simulink model "Final_Q2_C_end"  (R2019a)
settings: Solver=ode1  StartTime=0.0  StopTime=60  FixedStep=0.01  RelTol=1e-3  EnableMultiTasking=on
settings Model: Creator=enesu  LastModifiedBy=hp
settings SolverCC: AutoInsertRateTranBlk=on

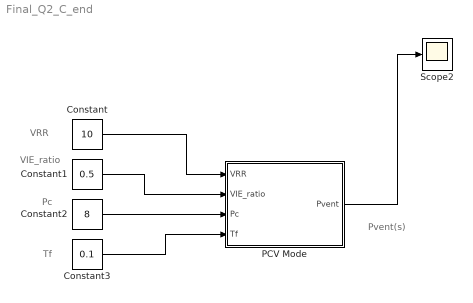
== system Final_Q2_C_end ==
  note: Tf
  note: Pc
  note: VIE_ratio
  note: VRR
  note: Pvent(s)
  Constant : Constant  Value=10  VectorParams1D=off
  Constant1 : Constant  Value=0.5
  Constant2 : Constant  Value=8
  Constant3 : Constant  Value=0.1
  PCV Mode : Subsystem
  Scope2 : Scope
  wires:
  Constant/1 -> PCV Mode/1(VRR)
  Constant1/1 -> PCV Mode/2(VIE_ratio)
  Constant2/1 -> PCV Mode/3(Pc)
  PCV Mode/1(Pvent) -> Scope2/1
  Constant3/1 -> PCV Mode/4(Tf)

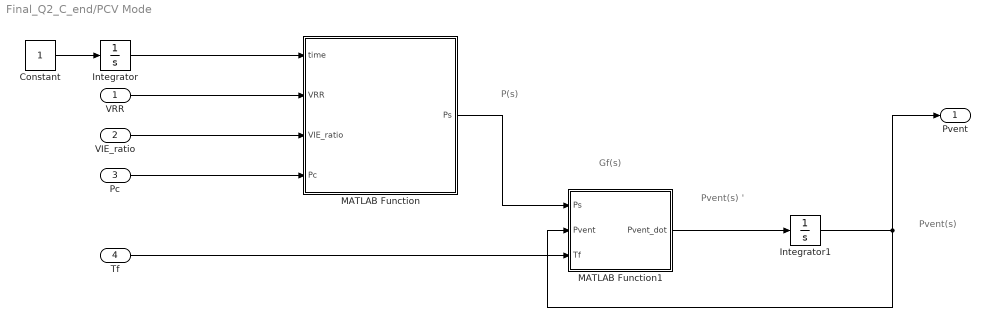
== system Final_Q2_C_end/PCV Mode ==
  note: P(s)
  note: Gf(s)
  note: Pvent(s) '
  note: Pvent(s)
  VRR : Inport
  VIE_ratio : Inport  Port=2
  Pc : Inport  Port=3
  Tf : Inport  Port=4
  Constant : Constant
  Integrator : Integrator
  Integrator1 : Integrator
  MATLAB Function : MATLAB Function  TreatAsAtomicUnit=on
  MATLAB Function1 : MATLAB Function  TreatAsAtomicUnit=on
  Pvent : Outport  VectorParamsAs1DForOutWhenUnconnected=on
  wires:
  Constant/1 -> Integrator/1
  Integrator/1 -> MATLAB Function/1(time)
  VRR/1 -> MATLAB Function/2(VRR)
  VIE_ratio/1 -> MATLAB Function/3(VIE_ratio)
  Pc/1 -> MATLAB Function/4(Pc)
  Tf/1 -> MATLAB Function1/3(Tf)
  MATLAB Function/1(Ps) -> MATLAB Function1/1(Ps)
  MATLAB Function1/1(Pvent_dot) -> Integrator1/1
  Integrator1/1 -> Pvent/1, MATLAB Function1/2(Pvent)

== matlab function Final_Q2_C_end/PCV Mode/MATLAB Function ==
  data: time input; Ps output; VRR input; VIE_ratio input; Pc input
function Ps = P_producer(time,VRR,VIE_ratio ,Pc)

stop_time = 60; % stop time is given as 60 seconds

% Ti - Inspiratory Time (s)     Te - Expiratory Time (s)
% VRR - Ventilator Respiratory Rate (breaths/min) is 10.
% VIE_ratio ventilator inspiratory/expiratory rate is 0.5.
% 
% There are 2 two equations.
%
%   60
% ------ = Ti + Te     and     Ti = Te x VIE
%   VRR
% 
% in matrix form;
%  _  _     _             _     _  _
% | 60 |   | 1      1      |   | Ti |
% | 0  | = | 1  -VIE_ratio | * | Te |
%  -  -     -             -     -  -
%
%   b = A.T 
%   T = inv(A).b

A = [ 1 1 ; 1 -VIE_ratio];
B = [stop_time/VRR ; 0];

T = inv(A)*B;

Ti = T(1); % Ti
Te = T(2); % Te



% We can set the period duration of the desired square wave 
% as [0, Ti + Te] by performing modulus operation.
time = mod(time , Ti + Te ); 

if( time <= Ti)
    Ps = Pc; 
else
    Ps = 0; 
end
end

== matlab function Final_Q2_C_end/PCV Mode/MATLAB Function1 ==
  data: Ps input; Pvent_dot output; Pvent input; Tf input
function Pvent_dot = filter(Ps,Pvent,Tf)
% Gf(s) = Pvent/ Ps = 1/( Tf*s + 1)
% Pvent* (Tf*s + 1) = Ps
% Pvent*Tf*s + Pvent = Ps
%
% In time domain 
% Pvent(t)' * Tf + Pvent(t) = P(t)
% Pvent(t)' = (P(t)  - Pvent(t))/ Tf
Pvent_dot = (Ps  - Pvent)/ Tf;

end
